simulink model "solved_LQR_observer"  (R2019a)
settings: Solver=ode45  StartTime=0.0  StopTime=simulation_time  MaxStep=0.01  RelTol=1e-3  EnableMultiTasking=on
values from neighbouring files (symbols this model uses):
  C = sol.updateCArray(Corig)    [exercise2_LQRandObserver.m]    (also in solEx1.m = eye(5); solEx2.m = eye(5))
  CObs = eye(5)    [solEx2.m]
  DObs = zeros(5,nObsState + nInputs)    [solEx2.m]
  L = place(Phi',c_meassurable',selected_poles)'    [solEx2.m]
  noiseMod = sol.getNoiseModule    [exercise2_LQRandObserver.m]
  parameters = sol.getSystemParameters    [exercise1_Linearization.m]    (also in exercise2_LQRandObserver.m; exercise3_DynamicProgramming.m; solEx1.m = zeros(5,1); solEx2.m = zeros(5,1))
  path_to_track = ut.genCircularPath(curvature)    [exercise1_Linearization.m]    (also in exercise3_DynamicProgramming.m = []; exercise4_NavigationFunction.m = [])
  Phi = Md.a    [solEx1.m]    (also in solEx2.m)
  sampling_time = 0.1    [exercise1_Linearization.m]    (also in exercise2_LQRandObserver.m = 0.01; exercise3_DynamicProgramming.m = 0.24)
  working_sensor = sol.getWorkingSensor    [exercise2_LQRandObserver.m]
  x0 = x0_experiments{exp_id}    [exercise1_Linearization.m]    (also in exercise3_DynamicProgramming.m = sol.getInitialState; solEx1.m = {x0_exp1, x0_exp2, x0_exp3, x0_exp3}; solEx2.m = [0, 0, 0, 0,0]'; solEx3.m = [20,1,0,0,0]')
  x0Obs = zeros(5,1)    [solEx2.m]
undefined symbols (not defined in the file or in its folder): Gam, lqr_gain
settings Model: Creator=ezequiel  LastModifiedBy=ezequiel
settings DataIOCC: ReturnWorkspaceOutputs=off
settings OptimizationCC: LifeSpan=inf
settings DebuggingCC: AllowSymbolicDim=off  PregeneratedLibrarySubsystemCodeDiagnostic=none  SFUnexpectedBacktrackingDiag=warning  SFNoUnconditionalDefaultTransitionDiag=warning  SFExecutionAtInitializationDiag=none  ArithmeticOperatorsInVariantConditions=warning
settings ModelReferenceCC: PropagateSignalLabelsOutOfModel=off
settings SFSimCC: SimUseLocalCustomCode=off
settings RTWCC: RTWUseLocalCustomCode=off
settings CodeAppCC: StateflowObjectComments=on
settings GRTTargetCC: TargetLangStandard=C89/C90 (ANSI)
settings ConfigComp: CovMetricSettings=dw  CovHtmlReporting=on  CovSaveCumulativeToWorkspaceVar=on  CovSaveSingleToWorkspaceVar=on  CovExternalEMLEnable=off

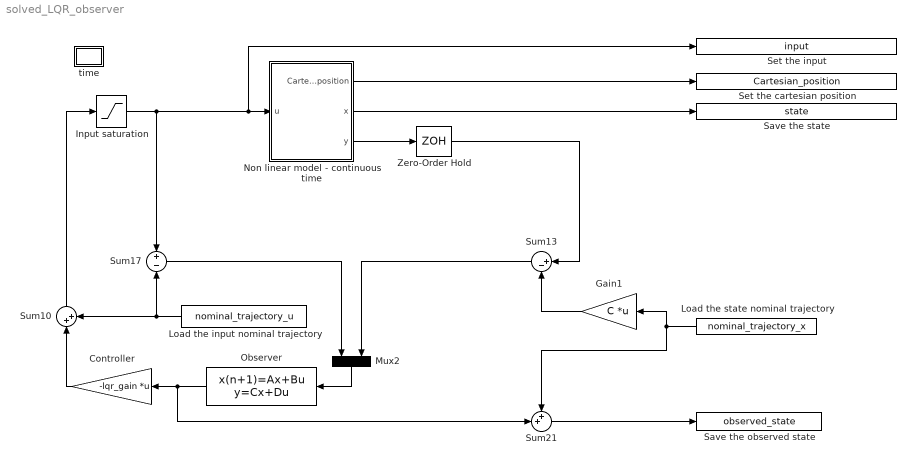
== system solved_LQR_observer ==
  Controller : Gain  Gain=-lqr_gain  Multiplication=Matrix(K*u)
  Gain1 : Gain  Gain=C  Multiplication=Matrix(K*u)
  Input saturation : Saturate  UpperLimit=[Inf;4*pi]  LowerLimit=[0;-4*pi]
  Load the input nominal trajectory : FromWorkspace  VariableName=nominal_trajectory_u  SampleTime=sampling_time  Interpolate=off  OutputAfterFinalValue=Holding final value
  Load the state nominal trajectory : FromWorkspace  VariableName=nominal_trajectory_x  SampleTime=sampling_time  Interpolate=off  OutputAfterFinalValue=Holding final value
  Mux2 : Mux  Inputs=2
  Non linear model - continuous time : Subsystem
  Observer : DiscreteStateSpace  A=Phi-L*C  B=[Gam L]  C=CObs  D=DObs  InitialCondition=x0Obs  SampleTime=sampling_time
  Save the observed state : ToWorkspace  VariableName=observed_state  SampleTime=-1
  Save the state : ToWorkspace  VariableName=state  SampleTime=-1
  Set the cartesian position : ToWorkspace  VariableName=Cartesian_position  SampleTime=-1
  Set the input : ToWorkspace  VariableName=input  SampleTime=-1
  Sum10 : Sum  Inputs=|++
  Sum13 : Sum  Inputs=|+-
  Sum17 : Sum  Inputs=+|-
  Sum21 : Sum  Inputs=++|
  Zero-Order Hold : ZeroOrderHold  SampleTime=sampling_time
  time : Subsystem
  wires:
  Load the state nominal trajectory/1 -> Sum21/1, Gain1/1
  Load the input nominal trajectory/1 -> Sum17/2, Sum10/2
  Sum10/1 -> Input saturation/1
  Observer/1 -> Sum21/2, Controller/1
  Sum13/1 -> Mux2/2
  Mux2/1 -> Observer/1
  Sum21/1 -> Save the observed state/1
  Input saturation/1 -> Sum17/1, Set the input/1, Non linear model - continuous time/1(u)
  Non linear model - continuous time/2(x) -> Save the state/1
  Non linear model - continuous time/3(y) -> Zero-Order Hold/1
  Non linear model - continuous time/1(Cartesian position) -> Set the cartesian position/1
  Zero-Order Hold/1 -> Sum13/1
  Gain1/1 -> Sum13/2
  Controller/1 -> Sum10/1
  Sum17/1 -> Mux2/1

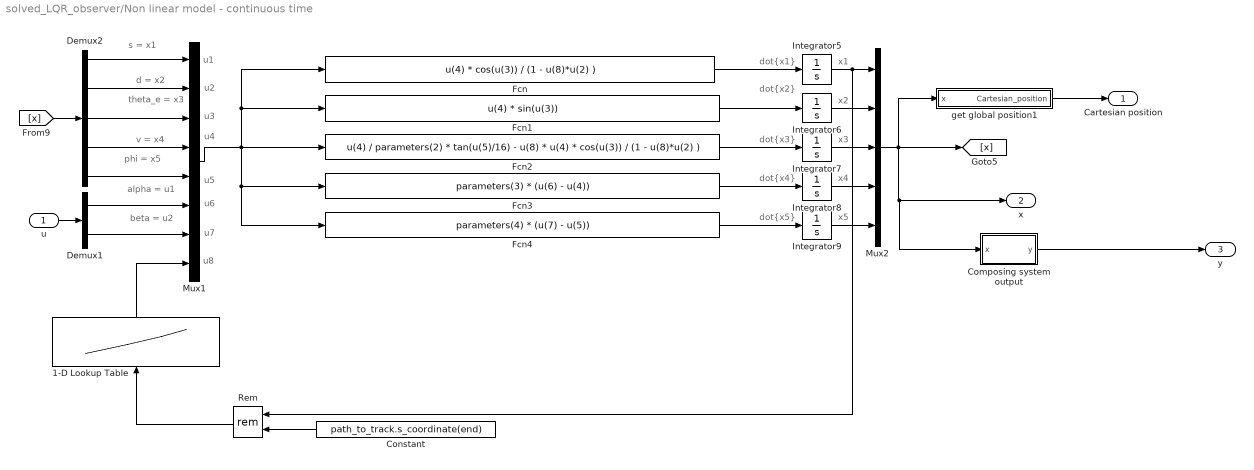
== system solved_LQR_observer/Non linear model - continuous time ==
  note: s = x1
  note: dot{x1}
  note: d = x2
  note: theta_e = x3
  note: v = x4
  note: phi = x5
  note: alpha = u1
  note: beta = u2
  note: u1
  note: u2
  note: u3
  note: u4
  note: u5
  note: u6
  note: u7
  note: x1
  note: dot{x2}
  note: x2
  note: dot{x3}
  note: x3
  note: dot{x4}
  note: x4
  note: dot{x5}
  note: x5
  note: u8
  u : Inport
  1-D Lookup Table : Lookup_n-D  NumberOfTableDimensions=1  BreakpointsForDimension1=path_to_track.s_coordinate  Table=path_to_track.curvature  InternalRulePriority=Speed  RndMeth=Simplest  InputSameDT=on
  Composing system output : Subsystem
  Constant : Constant  Value=path_to_track.s_coordinate(end)
  Demux1 : Demux  Outputs=2
  Demux2 : Demux  Outputs=5
  Fcn : Fcn  Expr=u(4) * cos(u(3)) / (1 - u(8)*u(2) )
  Fcn1 : Fcn  Expr=u(4) * sin(u(3))
  Fcn2 : Fcn  Expr=u(4) / parameters(2) * tan(u(5)/16) - u(8) * u(4) * cos(u(3)) / (1 - u(8)*u(2) )
  Fcn3 : Fcn  Expr=parameters(3) * (u(6) - u(4))
  Fcn4 : Fcn  Expr=parameters(4) * (u(7) - u(5))
  Integrator5 : Integrator  InitialCondition=x0(1)
  Integrator6 : Integrator  InitialCondition=x0(2)
  Integrator7 : Integrator  InitialCondition=x0(3)
  Integrator8 : Integrator  InitialCondition=x0(4)
  Integrator9 : Integrator  InitialCondition=x0(5)
  Mux1 : Mux  Inputs=8
  Mux2 : Mux  Inputs=5
  Rem : Math  Operator=rem  SaturateOnIntegerOverflow=on
  get global position1 : Subsystem
  Cartesian position : Outport
  x : Outport  Port=2
  y : Outport  Port=3
  wires:
  u/1 -> Demux1/1
  Fcn/1 -> Integrator5/1
  Demux2/1 -> Mux1/1
  Demux2/2 -> Mux1/2
  Demux2/3 -> Mux1/3
  Demux2/4 -> Mux1/4
  Demux2/5 -> Mux1/5
  Demux1/1 -> Mux1/6
  Demux1/2 -> Mux1/7
  Mux1/1 -> Fcn3/1, Fcn4/1, Fcn1/1, Fcn/1, Fcn2/1
  Fcn1/1 -> Integrator6/1
  Integrator6/1 -> Mux2/2
  Fcn2/1 -> Integrator7/1
  Integrator7/1 -> Mux2/3
  Fcn3/1 -> Integrator8/1
  Integrator8/1 -> Mux2/4
  Fcn4/1 -> Integrator9/1
  Integrator9/1 -> Mux2/5
  [x] -> Demux2/1
  1-D Lookup Table/1 -> Mux1/8
  Rem/1 -> 1-D Lookup Table/1
  Constant/1 -> Rem/2
  Integrator5/1 -> Rem/1, Mux2/1
  get global position1/1("Cartesian_position ") -> Cartesian position/1
  Mux2/1 -> get global position1/1(x), Composing system output/1(x), x/1, [x]
  Composing system output/1(y) -> y/1

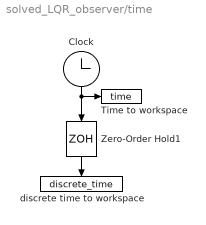
== system solved_LQR_observer/time ==
  Clock : Clock
  Time to workspace : ToWorkspace  VariableName=time  SampleTime=-1
  Zero-Order Hold1 : ZeroOrderHold  SampleTime=sampling_time
  discrete time to workspace : ToWorkspace  VariableName=discrete_time  SampleTime=-1
  wires:
  Clock/1 -> Zero-Order Hold1/1, Time to workspace/1
  Zero-Order Hold1/1 -> discrete time to workspace/1

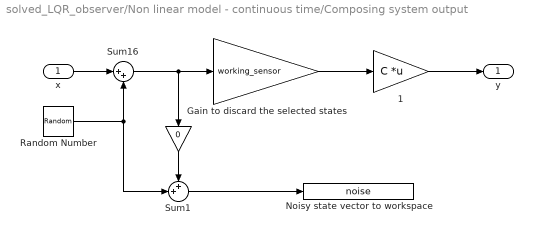
== system solved_LQR_observer/Non linear model - continuous time/Composing system output ==
  x : Inport
  " " : Gain  Gain=0
  " 1" : Gain  Gain=C  Multiplication=Matrix(K*u)
  Gain to discard the selected states : Gain  Gain=working_sensor
  Noisy state vector to workspace : ToWorkspace  VariableName=noise  SampleTime=-1
  Random Number : RandomNumber  Mean=noiseMod.mean  Variance=noiseMod.std_deviation.^2  Seed=noiseMod.seed  SampleTime=1/noiseMod.freq
  Sum1 : Sum  Inputs=++|
  Sum16 : Sum  Inputs=|++
  y : Outport
  wires:
  Gain to discard the selected states/1 -> " 1"/1
  Random Number/1 -> Sum1/2, Sum16/2
  Sum16/1 -> Gain to discard the selected states/1, " "/1
  Sum1/1 -> Noisy state vector to workspace/1
  x/1 -> Sum16/1
  " "/1 -> Sum1/1
  " 1"/1 -> y/1

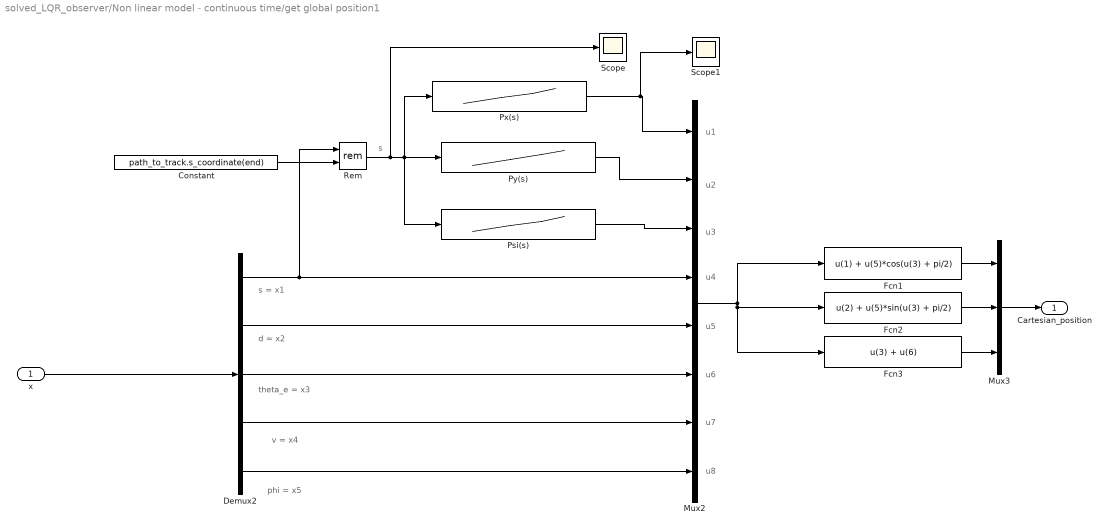
== system solved_LQR_observer/Non linear model - continuous time/get global position1 ==
  note: s
  note: s = x1
  note: d = x2
  note: theta_e = x3
  note: v = x4
  note: phi = x5
  note: u1
  note: u2
  note: u3
  note: u4
  note: u5
  note: u6
  note: u7
  note: u8
  x : Inport
  Constant : Constant  Value=path_to_track.s_coordinate(end)
  Demux2 : Demux  Outputs=5
  Fcn1 : Fcn  Expr=u(1) + u(5)*cos(u(3) + pi/2)
  Fcn2 : Fcn  Expr=u(2) + u(5)*sin(u(3) + pi/2)
  Fcn3 : Fcn  Expr=u(3) + u(6)
  Mux2 : Mux  Inputs=8
  Mux3 : Mux  Inputs=3
  Psi(s) : Lookup_n-D  NumberOfTableDimensions=1  BreakpointsForDimension1=path_to_track.s_coordinate  Table=path_to_track.orientation  InternalRulePriority=Speed  RndMeth=Simplest  InputSameDT=on
  Px(s) : Lookup_n-D  NumberOfTableDimensions=1  BreakpointsForDimension1=path_to_track.s_coordinate  Table=path_to_track.coordinates(:,1)  InternalRulePriority=Speed  RndMeth=Simplest  InputSameDT=on
  Py(s) : Lookup_n-D  NumberOfTableDimensions=1  BreakpointsForDimension1=path_to_track.s_coordinate  Table=path_to_track.coordinates(:,2)  InternalRulePriority=Speed  RndMeth=Simplest  InputSameDT=on
  Rem : Math  Operator=rem  SaturateOnIntegerOverflow=on
  Scope : Scope
  Scope1 : Scope
  "Cartesian_position " : Outport
  wires:
  Demux2/1 -> Mux2/4, Rem/1
  Mux3/1 -> "Cartesian_position "/1
  x/1 -> Demux2/1
  Rem/1 -> Scope/1, Psi(s)/1, Px(s)/1, Py(s)/1
  Constant/1 -> Rem/2
  Px(s)/1 -> Scope1/1, Mux2/1
  Py(s)/1 -> Mux2/2
  Psi(s)/1 -> Mux2/3
  Mux2/1 -> Fcn3/1, Fcn2/1, Fcn1/1
  Fcn1/1 -> Mux3/1
  Fcn2/1 -> Mux3/2
  Fcn3/1 -> Mux3/3
  Demux2/2 -> Mux2/5
  Demux2/3 -> Mux2/6
  Demux2/4 -> Mux2/7
  Demux2/5 -> Mux2/8
